simulink model "lab2_1"  (R2022a)
settings: Solver=FixedStepAuto  StartTime=0.0  StopTime=Tmdl  FixedStep=To/100  RelTol=1e-3
undefined symbols (not defined in the file or in its folder): an, dsc, To
settings Model: Creator=Professional  LastModifiedBy=osini

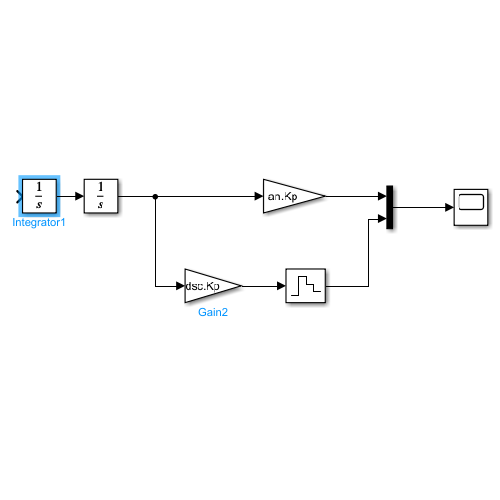
[thumbnail: Simulink's stored preview of the top-level diagram]
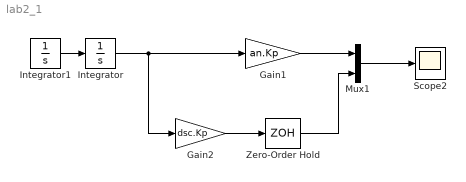
== system lab2_1 ==
  Gain1 : Gain  Gain=an.Kp
  Gain2 : Gain  Gain=dsc.Kp
  Integrator : Integrator
  Integrator1 : Integrator  InitialCondition=1
  Mux1 : Mux  Inputs=2
  Scope2 : Scope
  Zero-Order Hold : ZeroOrderHold  SampleTime=To
  wires:
  Gain1/1 -> Mux1/1
  Mux1/1 -> Scope2/1
  Integrator/1 -> Gain2/1, Gain1/1
  Gain2/1 -> Zero-Order Hold/1
  Zero-Order Hold/1 -> Mux1/2
  Integrator1/1 -> Integrator/1
